simulink model "Aloe_E_Cell_Project_2016"  (R2016b)
settings: Solver=VariableStepAuto  StartTime=0.0  StopTime=0.14  RelTol=1e-3
undefined symbols (not defined in the file): D1, Delta
libraries: powerlib x218, powerlib_meascontrol x6, simulink x2
(part 2 of 2)

== system Aloe_E_Cell_Project_2016/Aloe E Battery Array/12 V Aloe E-Cell26 ==
  Constant : Constant  Value=4
  Constant1 : Constant  Value=24
  Controlled Current Source : powerlib/Electrical Sources/Controlled Current Source  Initialize=on  Source_Type=DC  Amplitude=1  Phase=0  Frequency=0  Measurements=None
  Controlled Voltage Source : powerlib/Electrical Sources/Controlled Voltage Source  Initialize=on  Source_Type=DC  Amplitude=1  Phase=0  Frequency=0  Measurements=Voltage
  Current Measurement : powerlib/Measurements/Current Measurement  PhasorSimulation=off  OutputType=Complex  PSBequivalent=0
  Display : Display
      settings: Decimation=3
  Display1 : Display
      settings: Decimation=3
  Series RLC Branch1 : powerlib/Elements/Series RLC Branch  LConnTagsString=__new0  RConnTagsString=__new0  BranchType=R  Resistance=6  Inductance=1e-3  SetiL0=off  InitialCurrent=0  Capacitance=1e-6  Setx0=off  InitialVoltage=0  Measurements=None
  Voltage Measurement : powerlib/Measurements/Voltage Measurement  PhasorSimulation=off  OutputType=Complex  PSBequivalent=0
  V+ : PMIOPort  Side=Right
  "V- " : PMIOPort  Port=2  Side=Right
  wires:
  Constant/1 -> Controlled Current Source/1
  Constant1/1 -> Controlled Voltage Source/1
  Current Measurement/1 -> Display1/1
  Voltage Measurement/1 -> Display/1
  connections:
  Series RLC Branch1/LConn1 -- Current Measurement/RConn1 -- Voltage Measurement/LConn1 -- V+/RConn1
  Controlled Voltage Source/RConn1 -- Controlled Current Source/LConn1
  Controlled Voltage Source/LConn1 -- Series RLC Branch1/RConn1 -- Voltage Measurement/LConn2 -- "V- "/RConn1
  Controlled Current Source/RConn1 -- Current Measurement/LConn1

== system Aloe_E_Cell_Project_2016/Aloe E Battery Array/12 V Aloe E-Cell27 ==
  Constant : Constant  Value=4
  Constant1 : Constant  Value=24
  Controlled Current Source : powerlib/Electrical Sources/Controlled Current Source  Initialize=on  Source_Type=DC  Amplitude=1  Phase=0  Frequency=0  Measurements=None
  Controlled Voltage Source : powerlib/Electrical Sources/Controlled Voltage Source  Initialize=on  Source_Type=DC  Amplitude=1  Phase=0  Frequency=0  Measurements=Voltage
  Current Measurement : powerlib/Measurements/Current Measurement  PhasorSimulation=off  OutputType=Complex  PSBequivalent=0
  Display : Display
      settings: Decimation=3
  Display1 : Display
      settings: Decimation=3
  Series RLC Branch1 : powerlib/Elements/Series RLC Branch  LConnTagsString=__new0  RConnTagsString=__new0  BranchType=R  Resistance=6  Inductance=1e-3  SetiL0=off  InitialCurrent=0  Capacitance=1e-6  Setx0=off  InitialVoltage=0  Measurements=None
  Voltage Measurement : powerlib/Measurements/Voltage Measurement  PhasorSimulation=off  OutputType=Complex  PSBequivalent=0
  V+ : PMIOPort  Side=Right
  "V- " : PMIOPort  Port=2  Side=Right
  wires:
  Voltage Measurement/1 -> Display/1
  Current Measurement/1 -> Display1/1
  Constant1/1 -> Controlled Voltage Source/1
  Constant/1 -> Controlled Current Source/1
  connections:
  Controlled Current Source/RConn1 -- Current Measurement/LConn1
  "V- "/RConn1 -- Voltage Measurement/LConn2 -- Series RLC Branch1/RConn1 -- Controlled Voltage Source/LConn1
  Controlled Voltage Source/RConn1 -- Controlled Current Source/LConn1
  V+/RConn1 -- Voltage Measurement/LConn1 -- Current Measurement/RConn1 -- Series RLC Branch1/LConn1

== system Aloe_E_Cell_Project_2016/Aloe E Battery Array/12 V Aloe E-Cell28 ==
  Constant : Constant  Value=4
  Constant1 : Constant  Value=24
  Controlled Current Source : powerlib/Electrical Sources/Controlled Current Source  Initialize=on  Source_Type=DC  Amplitude=1  Phase=0  Frequency=0  Measurements=None
  Controlled Voltage Source : powerlib/Electrical Sources/Controlled Voltage Source  Initialize=on  Source_Type=DC  Amplitude=1  Phase=0  Frequency=0  Measurements=Voltage
  Current Measurement : powerlib/Measurements/Current Measurement  PhasorSimulation=off  OutputType=Complex  PSBequivalent=0
  Display : Display
      settings: Decimation=3
  Display1 : Display
      settings: Decimation=3
  Series RLC Branch1 : powerlib/Elements/Series RLC Branch  LConnTagsString=__new0  RConnTagsString=__new0  BranchType=R  Resistance=6  Inductance=1e-3  SetiL0=off  InitialCurrent=0  Capacitance=1e-6  Setx0=off  InitialVoltage=0  Measurements=None
  Voltage Measurement : powerlib/Measurements/Voltage Measurement  PhasorSimulation=off  OutputType=Complex  PSBequivalent=0
  V+ : PMIOPort  Side=Right
  "V- " : PMIOPort  Port=2  Side=Right
  wires:
  Voltage Measurement/1 -> Display/1
  Current Measurement/1 -> Display1/1
  Constant1/1 -> Controlled Voltage Source/1
  Constant/1 -> Controlled Current Source/1
  connections:
  Controlled Current Source/RConn1 -- Current Measurement/LConn1
  "V- "/RConn1 -- Voltage Measurement/LConn2 -- Series RLC Branch1/RConn1 -- Controlled Voltage Source/LConn1
  Controlled Voltage Source/RConn1 -- Controlled Current Source/LConn1
  V+/RConn1 -- Voltage Measurement/LConn1 -- Current Measurement/RConn1 -- Series RLC Branch1/LConn1

== system Aloe_E_Cell_Project_2016/Aloe E Battery Array/12 V Aloe E-Cell29 ==
  Constant : Constant  Value=4
  Constant1 : Constant  Value=24
  Controlled Current Source : powerlib/Electrical Sources/Controlled Current Source  Initialize=on  Source_Type=DC  Amplitude=1  Phase=0  Frequency=0  Measurements=None
  Controlled Voltage Source : powerlib/Electrical Sources/Controlled Voltage Source  Initialize=on  Source_Type=DC  Amplitude=1  Phase=0  Frequency=0  Measurements=Voltage
  Current Measurement : powerlib/Measurements/Current Measurement  PhasorSimulation=off  OutputType=Complex  PSBequivalent=0
  Display : Display
      settings: Decimation=3
  Display1 : Display
      settings: Decimation=3
  Series RLC Branch1 : powerlib/Elements/Series RLC Branch  LConnTagsString=__new0  RConnTagsString=__new0  BranchType=R  Resistance=6  Inductance=1e-3  SetiL0=off  InitialCurrent=0  Capacitance=1e-6  Setx0=off  InitialVoltage=0  Measurements=None
  Voltage Measurement : powerlib/Measurements/Voltage Measurement  PhasorSimulation=off  OutputType=Complex  PSBequivalent=0
  V+ : PMIOPort  Side=Right
  "V- " : PMIOPort  Port=2  Side=Right
  wires:
  Constant/1 -> Controlled Current Source/1
  Constant1/1 -> Controlled Voltage Source/1
  Current Measurement/1 -> Display1/1
  Voltage Measurement/1 -> Display/1
  connections:
  Series RLC Branch1/LConn1 -- Current Measurement/RConn1 -- Voltage Measurement/LConn1 -- V+/RConn1
  Controlled Voltage Source/RConn1 -- Controlled Current Source/LConn1
  Controlled Voltage Source/LConn1 -- Series RLC Branch1/RConn1 -- Voltage Measurement/LConn2 -- "V- "/RConn1
  Controlled Current Source/RConn1 -- Current Measurement/LConn1

== system Aloe_E_Cell_Project_2016/Aloe E Battery Array/12 V Aloe E-Cell3 ==
  Constant : Constant  Value=4
  Constant1 : Constant  Value=24
  Controlled Current Source : powerlib/Electrical Sources/Controlled Current Source  Initialize=on  Source_Type=DC  Amplitude=1  Phase=0  Frequency=0  Measurements=None
  Controlled Voltage Source : powerlib/Electrical Sources/Controlled Voltage Source  Initialize=on  Source_Type=DC  Amplitude=1  Phase=0  Frequency=0  Measurements=Voltage
  Current Measurement : powerlib/Measurements/Current Measurement  PhasorSimulation=off  OutputType=Complex  PSBequivalent=0
  Display : Display
      settings: Decimation=3
  Display1 : Display
      settings: Decimation=3
  Series RLC Branch1 : powerlib/Elements/Series RLC Branch  LConnTagsString=__new0  RConnTagsString=__new0  BranchType=R  Resistance=6  Inductance=1e-3  SetiL0=off  InitialCurrent=0  Capacitance=1e-6  Setx0=off  InitialVoltage=0  Measurements=None
  Voltage Measurement : powerlib/Measurements/Voltage Measurement  PhasorSimulation=off  OutputType=Complex  PSBequivalent=0
  V+ : PMIOPort  Side=Right
  "V- " : PMIOPort  Port=2  Side=Right
  wires:
  Constant/1 -> Controlled Current Source/1
  Constant1/1 -> Controlled Voltage Source/1
  Current Measurement/1 -> Display1/1
  Voltage Measurement/1 -> Display/1
  connections:
  Series RLC Branch1/LConn1 -- Current Measurement/RConn1 -- Voltage Measurement/LConn1 -- V+/RConn1
  Controlled Voltage Source/RConn1 -- Controlled Current Source/LConn1
  Controlled Voltage Source/LConn1 -- Series RLC Branch1/RConn1 -- Voltage Measurement/LConn2 -- "V- "/RConn1
  Controlled Current Source/RConn1 -- Current Measurement/LConn1

== system Aloe_E_Cell_Project_2016/Aloe E Battery Array/12 V Aloe E-Cell30 ==
  Constant : Constant  Value=4
  Constant1 : Constant  Value=24
  Controlled Current Source : powerlib/Electrical Sources/Controlled Current Source  Initialize=on  Source_Type=DC  Amplitude=1  Phase=0  Frequency=0  Measurements=None
  Controlled Voltage Source : powerlib/Electrical Sources/Controlled Voltage Source  Initialize=on  Source_Type=DC  Amplitude=1  Phase=0  Frequency=0  Measurements=Voltage
  Current Measurement : powerlib/Measurements/Current Measurement  PhasorSimulation=off  OutputType=Complex  PSBequivalent=0
  Display : Display
      settings: Decimation=3
  Display1 : Display
      settings: Decimation=3
  Series RLC Branch1 : powerlib/Elements/Series RLC Branch  LConnTagsString=__new0  RConnTagsString=__new0  BranchType=R  Resistance=6  Inductance=1e-3  SetiL0=off  InitialCurrent=0  Capacitance=1e-6  Setx0=off  InitialVoltage=0  Measurements=None
  Voltage Measurement : powerlib/Measurements/Voltage Measurement  PhasorSimulation=off  OutputType=Complex  PSBequivalent=0
  V+ : PMIOPort  Side=Right
  "V- " : PMIOPort  Port=2  Side=Right
  wires:
  Constant/1 -> Controlled Current Source/1
  Constant1/1 -> Controlled Voltage Source/1
  Current Measurement/1 -> Display1/1
  Voltage Measurement/1 -> Display/1
  connections:
  Series RLC Branch1/LConn1 -- Current Measurement/RConn1 -- Voltage Measurement/LConn1 -- V+/RConn1
  Controlled Voltage Source/RConn1 -- Controlled Current Source/LConn1
  Controlled Voltage Source/LConn1 -- Series RLC Branch1/RConn1 -- Voltage Measurement/LConn2 -- "V- "/RConn1
  Controlled Current Source/RConn1 -- Current Measurement/LConn1

== system Aloe_E_Cell_Project_2016/Aloe E Battery Array/12 V Aloe E-Cell31 ==
  Constant : Constant  Value=4
  Constant1 : Constant  Value=24
  Controlled Current Source : powerlib/Electrical Sources/Controlled Current Source  Initialize=on  Source_Type=DC  Amplitude=1  Phase=0  Frequency=0  Measurements=None
  Controlled Voltage Source : powerlib/Electrical Sources/Controlled Voltage Source  Initialize=on  Source_Type=DC  Amplitude=1  Phase=0  Frequency=0  Measurements=Voltage
  Current Measurement : powerlib/Measurements/Current Measurement  PhasorSimulation=off  OutputType=Complex  PSBequivalent=0
  Display : Display
      settings: Decimation=3
  Display1 : Display
      settings: Decimation=3
  Series RLC Branch1 : powerlib/Elements/Series RLC Branch  LConnTagsString=__new0  RConnTagsString=__new0  BranchType=R  Resistance=6  Inductance=1e-3  SetiL0=off  InitialCurrent=0  Capacitance=1e-6  Setx0=off  InitialVoltage=0  Measurements=None
  Voltage Measurement : powerlib/Measurements/Voltage Measurement  PhasorSimulation=off  OutputType=Complex  PSBequivalent=0
  V+ : PMIOPort  Side=Right
  "V- " : PMIOPort  Port=2  Side=Right
  wires:
  Voltage Measurement/1 -> Display/1
  Current Measurement/1 -> Display1/1
  Constant1/1 -> Controlled Voltage Source/1
  Constant/1 -> Controlled Current Source/1
  connections:
  Controlled Current Source/RConn1 -- Current Measurement/LConn1
  "V- "/RConn1 -- Voltage Measurement/LConn2 -- Series RLC Branch1/RConn1 -- Controlled Voltage Source/LConn1
  Controlled Voltage Source/RConn1 -- Controlled Current Source/LConn1
  V+/RConn1 -- Voltage Measurement/LConn1 -- Current Measurement/RConn1 -- Series RLC Branch1/LConn1

== system Aloe_E_Cell_Project_2016/Aloe E Battery Array/12 V Aloe E-Cell32 ==
  Constant : Constant  Value=4
  Constant1 : Constant  Value=24
  Controlled Current Source : powerlib/Electrical Sources/Controlled Current Source  Initialize=on  Source_Type=DC  Amplitude=1  Phase=0  Frequency=0  Measurements=None
  Controlled Voltage Source : powerlib/Electrical Sources/Controlled Voltage Source  Initialize=on  Source_Type=DC  Amplitude=1  Phase=0  Frequency=0  Measurements=Voltage
  Current Measurement : powerlib/Measurements/Current Measurement  PhasorSimulation=off  OutputType=Complex  PSBequivalent=0
  Display : Display
      settings: Decimation=3
  Display1 : Display
      settings: Decimation=3
  Series RLC Branch1 : powerlib/Elements/Series RLC Branch  LConnTagsString=__new0  RConnTagsString=__new0  BranchType=R  Resistance=6  Inductance=1e-3  SetiL0=off  InitialCurrent=0  Capacitance=1e-6  Setx0=off  InitialVoltage=0  Measurements=None
  Voltage Measurement : powerlib/Measurements/Voltage Measurement  PhasorSimulation=off  OutputType=Complex  PSBequivalent=0
  V+ : PMIOPort  Side=Right
  "V- " : PMIOPort  Port=2  Side=Right
  wires:
  Constant/1 -> Controlled Current Source/1
  Constant1/1 -> Controlled Voltage Source/1
  Current Measurement/1 -> Display1/1
  Voltage Measurement/1 -> Display/1
  connections:
  Series RLC Branch1/LConn1 -- Current Measurement/RConn1 -- Voltage Measurement/LConn1 -- V+/RConn1
  Controlled Voltage Source/RConn1 -- Controlled Current Source/LConn1
  Controlled Voltage Source/LConn1 -- Series RLC Branch1/RConn1 -- Voltage Measurement/LConn2 -- "V- "/RConn1
  Controlled Current Source/RConn1 -- Current Measurement/LConn1

== system Aloe_E_Cell_Project_2016/Aloe E Battery Array/12 V Aloe E-Cell33 ==
  Constant : Constant  Value=4
  Constant1 : Constant  Value=24
  Controlled Current Source : powerlib/Electrical Sources/Controlled Current Source  Initialize=on  Source_Type=DC  Amplitude=1  Phase=0  Frequency=0  Measurements=None
  Controlled Voltage Source : powerlib/Electrical Sources/Controlled Voltage Source  Initialize=on  Source_Type=DC  Amplitude=1  Phase=0  Frequency=0  Measurements=Voltage
  Current Measurement : powerlib/Measurements/Current Measurement  PhasorSimulation=off  OutputType=Complex  PSBequivalent=0
  Display : Display
      settings: Decimation=3
  Display1 : Display
      settings: Decimation=3
  Series RLC Branch1 : powerlib/Elements/Series RLC Branch  LConnTagsString=__new0  RConnTagsString=__new0  BranchType=R  Resistance=6  Inductance=1e-3  SetiL0=off  InitialCurrent=0  Capacitance=1e-6  Setx0=off  InitialVoltage=0  Measurements=None
  Voltage Measurement : powerlib/Measurements/Voltage Measurement  PhasorSimulation=off  OutputType=Complex  PSBequivalent=0
  V+ : PMIOPort  Side=Right
  "V- " : PMIOPort  Port=2  Side=Right
  wires:
  Constant/1 -> Controlled Current Source/1
  Constant1/1 -> Controlled Voltage Source/1
  Current Measurement/1 -> Display1/1
  Voltage Measurement/1 -> Display/1
  connections:
  Series RLC Branch1/LConn1 -- Current Measurement/RConn1 -- Voltage Measurement/LConn1 -- V+/RConn1
  Controlled Voltage Source/RConn1 -- Controlled Current Source/LConn1
  Controlled Voltage Source/LConn1 -- Series RLC Branch1/RConn1 -- Voltage Measurement/LConn2 -- "V- "/RConn1
  Controlled Current Source/RConn1 -- Current Measurement/LConn1

== system Aloe_E_Cell_Project_2016/Aloe E Battery Array/12 V Aloe E-Cell34 ==
  Constant : Constant  Value=4
  Constant1 : Constant  Value=24
  Controlled Current Source : powerlib/Electrical Sources/Controlled Current Source  Initialize=on  Source_Type=DC  Amplitude=1  Phase=0  Frequency=0  Measurements=None
  Controlled Voltage Source : powerlib/Electrical Sources/Controlled Voltage Source  Initialize=on  Source_Type=DC  Amplitude=1  Phase=0  Frequency=0  Measurements=Voltage
  Current Measurement : powerlib/Measurements/Current Measurement  PhasorSimulation=off  OutputType=Complex  PSBequivalent=0
  Display : Display
      settings: Decimation=3
  Display1 : Display
      settings: Decimation=3
  Series RLC Branch1 : powerlib/Elements/Series RLC Branch  LConnTagsString=__new0  RConnTagsString=__new0  BranchType=R  Resistance=6  Inductance=1e-3  SetiL0=off  InitialCurrent=0  Capacitance=1e-6  Setx0=off  InitialVoltage=0  Measurements=None
  Voltage Measurement : powerlib/Measurements/Voltage Measurement  PhasorSimulation=off  OutputType=Complex  PSBequivalent=0
  V+ : PMIOPort  Side=Right
  "V- " : PMIOPort  Port=2  Side=Right
  wires:
  Voltage Measurement/1 -> Display/1
  Current Measurement/1 -> Display1/1
  Constant1/1 -> Controlled Voltage Source/1
  Constant/1 -> Controlled Current Source/1
  connections:
  Controlled Current Source/RConn1 -- Current Measurement/LConn1
  "V- "/RConn1 -- Voltage Measurement/LConn2 -- Series RLC Branch1/RConn1 -- Controlled Voltage Source/LConn1
  Controlled Voltage Source/RConn1 -- Controlled Current Source/LConn1
  V+/RConn1 -- Voltage Measurement/LConn1 -- Current Measurement/RConn1 -- Series RLC Branch1/LConn1

== system Aloe_E_Cell_Project_2016/Aloe E Battery Array/12 V Aloe E-Cell35 ==
  Constant : Constant  Value=4
  Constant1 : Constant  Value=24
  Controlled Current Source : powerlib/Electrical Sources/Controlled Current Source  Initialize=on  Source_Type=DC  Amplitude=1  Phase=0  Frequency=0  Measurements=None
  Controlled Voltage Source : powerlib/Electrical Sources/Controlled Voltage Source  Initialize=on  Source_Type=DC  Amplitude=1  Phase=0  Frequency=0  Measurements=Voltage
  Current Measurement : powerlib/Measurements/Current Measurement  PhasorSimulation=off  OutputType=Complex  PSBequivalent=0
  Display : Display
      settings: Decimation=3
  Display1 : Display
      settings: Decimation=3
  Series RLC Branch1 : powerlib/Elements/Series RLC Branch  LConnTagsString=__new0  RConnTagsString=__new0  BranchType=R  Resistance=6  Inductance=1e-3  SetiL0=off  InitialCurrent=0  Capacitance=1e-6  Setx0=off  InitialVoltage=0  Measurements=None
  Voltage Measurement : powerlib/Measurements/Voltage Measurement  PhasorSimulation=off  OutputType=Complex  PSBequivalent=0
  V+ : PMIOPort  Side=Right
  "V- " : PMIOPort  Port=2  Side=Right
  wires:
  Constant/1 -> Controlled Current Source/1
  Constant1/1 -> Controlled Voltage Source/1
  Current Measurement/1 -> Display1/1
  Voltage Measurement/1 -> Display/1
  connections:
  Series RLC Branch1/LConn1 -- Current Measurement/RConn1 -- Voltage Measurement/LConn1 -- V+/RConn1
  Controlled Voltage Source/RConn1 -- Controlled Current Source/LConn1
  Controlled Voltage Source/LConn1 -- Series RLC Branch1/RConn1 -- Voltage Measurement/LConn2 -- "V- "/RConn1
  Controlled Current Source/RConn1 -- Current Measurement/LConn1

== system Aloe_E_Cell_Project_2016/Aloe E Battery Array/12 V Aloe E-Cell36 ==
  Constant : Constant  Value=4
  Constant1 : Constant  Value=24
  Controlled Current Source : powerlib/Electrical Sources/Controlled Current Source  Initialize=on  Source_Type=DC  Amplitude=1  Phase=0  Frequency=0  Measurements=None
  Controlled Voltage Source : powerlib/Electrical Sources/Controlled Voltage Source  Initialize=on  Source_Type=DC  Amplitude=1  Phase=0  Frequency=0  Measurements=Voltage
  Current Measurement : powerlib/Measurements/Current Measurement  PhasorSimulation=off  OutputType=Complex  PSBequivalent=0
  Display : Display
      settings: Decimation=3
  Display1 : Display
      settings: Decimation=3
  Series RLC Branch1 : powerlib/Elements/Series RLC Branch  LConnTagsString=__new0  RConnTagsString=__new0  BranchType=R  Resistance=6  Inductance=1e-3  SetiL0=off  InitialCurrent=0  Capacitance=1e-6  Setx0=off  InitialVoltage=0  Measurements=None
  Voltage Measurement : powerlib/Measurements/Voltage Measurement  PhasorSimulation=off  OutputType=Complex  PSBequivalent=0
  V+ : PMIOPort  Side=Right
  "V- " : PMIOPort  Port=2  Side=Right
  wires:
  Constant/1 -> Controlled Current Source/1
  Constant1/1 -> Controlled Voltage Source/1
  Current Measurement/1 -> Display1/1
  Voltage Measurement/1 -> Display/1
  connections:
  Series RLC Branch1/LConn1 -- Current Measurement/RConn1 -- Voltage Measurement/LConn1 -- V+/RConn1
  Controlled Voltage Source/RConn1 -- Controlled Current Source/LConn1
  Controlled Voltage Source/LConn1 -- Series RLC Branch1/RConn1 -- Voltage Measurement/LConn2 -- "V- "/RConn1
  Controlled Current Source/RConn1 -- Current Measurement/LConn1

== system Aloe_E_Cell_Project_2016/Aloe E Battery Array/12 V Aloe E-Cell37 ==
  Constant : Constant  Value=4
  Constant1 : Constant  Value=24
  Controlled Current Source : powerlib/Electrical Sources/Controlled Current Source  Initialize=on  Source_Type=DC  Amplitude=1  Phase=0  Frequency=0  Measurements=None
  Controlled Voltage Source : powerlib/Electrical Sources/Controlled Voltage Source  Initialize=on  Source_Type=DC  Amplitude=1  Phase=0  Frequency=0  Measurements=Voltage
  Current Measurement : powerlib/Measurements/Current Measurement  PhasorSimulation=off  OutputType=Complex  PSBequivalent=0
  Display : Display
      settings: Decimation=3
  Display1 : Display
      settings: Decimation=3
  Series RLC Branch1 : powerlib/Elements/Series RLC Branch  LConnTagsString=__new0  RConnTagsString=__new0  BranchType=R  Resistance=6  Inductance=1e-3  SetiL0=off  InitialCurrent=0  Capacitance=1e-6  Setx0=off  InitialVoltage=0  Measurements=None
  Voltage Measurement : powerlib/Measurements/Voltage Measurement  PhasorSimulation=off  OutputType=Complex  PSBequivalent=0
  V+ : PMIOPort  Side=Right
  "V- " : PMIOPort  Port=2  Side=Right
  wires:
  Voltage Measurement/1 -> Display/1
  Current Measurement/1 -> Display1/1
  Constant1/1 -> Controlled Voltage Source/1
  Constant/1 -> Controlled Current Source/1
  connections:
  Controlled Current Source/RConn1 -- Current Measurement/LConn1
  "V- "/RConn1 -- Voltage Measurement/LConn2 -- Series RLC Branch1/RConn1 -- Controlled Voltage Source/LConn1
  Controlled Voltage Source/RConn1 -- Controlled Current Source/LConn1
  V+/RConn1 -- Voltage Measurement/LConn1 -- Current Measurement/RConn1 -- Series RLC Branch1/LConn1

== system Aloe_E_Cell_Project_2016/Aloe E Battery Array/12 V Aloe E-Cell38 ==
  Constant : Constant  Value=4
  Constant1 : Constant  Value=24
  Controlled Current Source : powerlib/Electrical Sources/Controlled Current Source  Initialize=on  Source_Type=DC  Amplitude=1  Phase=0  Frequency=0  Measurements=None
  Controlled Voltage Source : powerlib/Electrical Sources/Controlled Voltage Source  Initialize=on  Source_Type=DC  Amplitude=1  Phase=0  Frequency=0  Measurements=Voltage
  Current Measurement : powerlib/Measurements/Current Measurement  PhasorSimulation=off  OutputType=Complex  PSBequivalent=0
  Display : Display
      settings: Decimation=3
  Display1 : Display
      settings: Decimation=3
  Series RLC Branch1 : powerlib/Elements/Series RLC Branch  LConnTagsString=__new0  RConnTagsString=__new0  BranchType=R  Resistance=6  Inductance=1e-3  SetiL0=off  InitialCurrent=0  Capacitance=1e-6  Setx0=off  InitialVoltage=0  Measurements=None
  Voltage Measurement : powerlib/Measurements/Voltage Measurement  PhasorSimulation=off  OutputType=Complex  PSBequivalent=0
  V+ : PMIOPort  Side=Right
  "V- " : PMIOPort  Port=2  Side=Right
  wires:
  Voltage Measurement/1 -> Display/1
  Current Measurement/1 -> Display1/1
  Constant1/1 -> Controlled Voltage Source/1
  Constant/1 -> Controlled Current Source/1
  connections:
  Controlled Current Source/RConn1 -- Current Measurement/LConn1
  "V- "/RConn1 -- Voltage Measurement/LConn2 -- Series RLC Branch1/RConn1 -- Controlled Voltage Source/LConn1
  Controlled Voltage Source/RConn1 -- Controlled Current Source/LConn1
  V+/RConn1 -- Voltage Measurement/LConn1 -- Current Measurement/RConn1 -- Series RLC Branch1/LConn1

== system Aloe_E_Cell_Project_2016/Aloe E Battery Array/12 V Aloe E-Cell39 ==
  Constant : Constant  Value=4
  Constant1 : Constant  Value=24
  Controlled Current Source : powerlib/Electrical Sources/Controlled Current Source  Initialize=on  Source_Type=DC  Amplitude=1  Phase=0  Frequency=0  Measurements=None
  Controlled Voltage Source : powerlib/Electrical Sources/Controlled Voltage Source  Initialize=on  Source_Type=DC  Amplitude=1  Phase=0  Frequency=0  Measurements=Voltage
  Current Measurement : powerlib/Measurements/Current Measurement  PhasorSimulation=off  OutputType=Complex  PSBequivalent=0
  Display : Display
      settings: Decimation=3
  Display1 : Display
      settings: Decimation=3
  Series RLC Branch1 : powerlib/Elements/Series RLC Branch  LConnTagsString=__new0  RConnTagsString=__new0  BranchType=R  Resistance=6  Inductance=1e-3  SetiL0=off  InitialCurrent=0  Capacitance=1e-6  Setx0=off  InitialVoltage=0  Measurements=None
  Voltage Measurement : powerlib/Measurements/Voltage Measurement  PhasorSimulation=off  OutputType=Complex  PSBequivalent=0
  V+ : PMIOPort  Side=Right
  "V- " : PMIOPort  Port=2  Side=Right
  wires:
  Constant/1 -> Controlled Current Source/1
  Constant1/1 -> Controlled Voltage Source/1
  Current Measurement/1 -> Display1/1
  Voltage Measurement/1 -> Display/1
  connections:
  Series RLC Branch1/LConn1 -- Current Measurement/RConn1 -- Voltage Measurement/LConn1 -- V+/RConn1
  Controlled Voltage Source/RConn1 -- Controlled Current Source/LConn1
  Controlled Voltage Source/LConn1 -- Series RLC Branch1/RConn1 -- Voltage Measurement/LConn2 -- "V- "/RConn1
  Controlled Current Source/RConn1 -- Current Measurement/LConn1

== system Aloe_E_Cell_Project_2016/Aloe E Battery Array/12 V Aloe E-Cell4 ==
  Constant : Constant  Value=4
  Constant1 : Constant  Value=24
  Controlled Current Source : powerlib/Electrical Sources/Controlled Current Source  Initialize=on  Source_Type=DC  Amplitude=1  Phase=0  Frequency=0  Measurements=None
  Controlled Voltage Source : powerlib/Electrical Sources/Controlled Voltage Source  Initialize=on  Source_Type=DC  Amplitude=1  Phase=0  Frequency=0  Measurements=Voltage
  Current Measurement : powerlib/Measurements/Current Measurement  PhasorSimulation=off  OutputType=Complex  PSBequivalent=0
  Display : Display
      settings: Decimation=3
  Display1 : Display
      settings: Decimation=3
  Series RLC Branch1 : powerlib/Elements/Series RLC Branch  LConnTagsString=__new0  RConnTagsString=__new0  BranchType=R  Resistance=6  Inductance=1e-3  SetiL0=off  InitialCurrent=0  Capacitance=1e-6  Setx0=off  InitialVoltage=0  Measurements=None
  Voltage Measurement : powerlib/Measurements/Voltage Measurement  PhasorSimulation=off  OutputType=Complex  PSBequivalent=0
  V+ : PMIOPort  Side=Right
  "V- " : PMIOPort  Port=2  Side=Right
  wires:
  Voltage Measurement/1 -> Display/1
  Current Measurement/1 -> Display1/1
  Constant1/1 -> Controlled Voltage Source/1
  Constant/1 -> Controlled Current Source/1
  connections:
  Controlled Current Source/RConn1 -- Current Measurement/LConn1
  "V- "/RConn1 -- Voltage Measurement/LConn2 -- Series RLC Branch1/RConn1 -- Controlled Voltage Source/LConn1
  Controlled Voltage Source/RConn1 -- Controlled Current Source/LConn1
  V+/RConn1 -- Voltage Measurement/LConn1 -- Current Measurement/RConn1 -- Series RLC Branch1/LConn1

== system Aloe_E_Cell_Project_2016/Aloe E Battery Array/12 V Aloe E-Cell40 ==
  Constant : Constant  Value=4
  Constant1 : Constant  Value=24
  Controlled Current Source : powerlib/Electrical Sources/Controlled Current Source  Initialize=on  Source_Type=DC  Amplitude=1  Phase=0  Frequency=0  Measurements=None
  Controlled Voltage Source : powerlib/Electrical Sources/Controlled Voltage Source  Initialize=on  Source_Type=DC  Amplitude=1  Phase=0  Frequency=0  Measurements=Voltage
  Current Measurement : powerlib/Measurements/Current Measurement  PhasorSimulation=off  OutputType=Complex  PSBequivalent=0
  Display : Display
      settings: Decimation=3
  Display1 : Display
      settings: Decimation=3
  Series RLC Branch1 : powerlib/Elements/Series RLC Branch  LConnTagsString=__new0  RConnTagsString=__new0  BranchType=R  Resistance=6  Inductance=1e-3  SetiL0=off  InitialCurrent=0  Capacitance=1e-6  Setx0=off  InitialVoltage=0  Measurements=None
  Voltage Measurement : powerlib/Measurements/Voltage Measurement  PhasorSimulation=off  OutputType=Complex  PSBequivalent=0
  V+ : PMIOPort  Side=Right
  "V- " : PMIOPort  Port=2  Side=Right
  wires:
  Voltage Measurement/1 -> Display/1
  Current Measurement/1 -> Display1/1
  Constant1/1 -> Controlled Voltage Source/1
  Constant/1 -> Controlled Current Source/1
  connections:
  Controlled Current Source/RConn1 -- Current Measurement/LConn1
  "V- "/RConn1 -- Voltage Measurement/LConn2 -- Series RLC Branch1/RConn1 -- Controlled Voltage Source/LConn1
  Controlled Voltage Source/RConn1 -- Controlled Current Source/LConn1
  V+/RConn1 -- Voltage Measurement/LConn1 -- Current Measurement/RConn1 -- Series RLC Branch1/LConn1

== system Aloe_E_Cell_Project_2016/Aloe E Battery Array/12 V Aloe E-Cell5 ==
  Constant : Constant  Value=4
  Constant1 : Constant  Value=24
  Controlled Current Source : powerlib/Electrical Sources/Controlled Current Source  Initialize=on  Source_Type=DC  Amplitude=1  Phase=0  Frequency=0  Measurements=None
  Controlled Voltage Source : powerlib/Electrical Sources/Controlled Voltage Source  Initialize=on  Source_Type=DC  Amplitude=1  Phase=0  Frequency=0  Measurements=Voltage
  Current Measurement : powerlib/Measurements/Current Measurement  PhasorSimulation=off  OutputType=Complex  PSBequivalent=0
  Display : Display
      settings: Decimation=3
  Display1 : Display
      settings: Decimation=3
  Series RLC Branch1 : powerlib/Elements/Series RLC Branch  LConnTagsString=__new0  RConnTagsString=__new0  BranchType=R  Resistance=6  Inductance=1e-3  SetiL0=off  InitialCurrent=0  Capacitance=1e-6  Setx0=off  InitialVoltage=0  Measurements=None
  Voltage Measurement : powerlib/Measurements/Voltage Measurement  PhasorSimulation=off  OutputType=Complex  PSBequivalent=0
  V+ : PMIOPort  Side=Right
  "V- " : PMIOPort  Port=2  Side=Right
  wires:
  Voltage Measurement/1 -> Display/1
  Current Measurement/1 -> Display1/1
  Constant1/1 -> Controlled Voltage Source/1
  Constant/1 -> Controlled Current Source/1
  connections:
  Controlled Current Source/RConn1 -- Current Measurement/LConn1
  "V- "/RConn1 -- Voltage Measurement/LConn2 -- Series RLC Branch1/RConn1 -- Controlled Voltage Source/LConn1
  Controlled Voltage Source/RConn1 -- Controlled Current Source/LConn1
  V+/RConn1 -- Voltage Measurement/LConn1 -- Current Measurement/RConn1 -- Series RLC Branch1/LConn1

== system Aloe_E_Cell_Project_2016/Aloe E Battery Array/12 V Aloe E-Cell6 ==
  Constant : Constant  Value=4
  Constant1 : Constant  Value=24
  Controlled Current Source : powerlib/Electrical Sources/Controlled Current Source  Initialize=on  Source_Type=DC  Amplitude=1  Phase=0  Frequency=0  Measurements=None
  Controlled Voltage Source : powerlib/Electrical Sources/Controlled Voltage Source  Initialize=on  Source_Type=DC  Amplitude=1  Phase=0  Frequency=0  Measurements=Voltage
  Current Measurement : powerlib/Measurements/Current Measurement  PhasorSimulation=off  OutputType=Complex  PSBequivalent=0
  Display : Display
      settings: Decimation=3
  Display1 : Display
      settings: Decimation=3
  Series RLC Branch1 : powerlib/Elements/Series RLC Branch  LConnTagsString=__new0  RConnTagsString=__new0  BranchType=R  Resistance=6  Inductance=1e-3  SetiL0=off  InitialCurrent=0  Capacitance=1e-6  Setx0=off  InitialVoltage=0  Measurements=None
  Voltage Measurement : powerlib/Measurements/Voltage Measurement  PhasorSimulation=off  OutputType=Complex  PSBequivalent=0
  V+ : PMIOPort  Side=Right
  "V- " : PMIOPort  Port=2  Side=Right
  wires:
  Constant/1 -> Controlled Current Source/1
  Constant1/1 -> Controlled Voltage Source/1
  Current Measurement/1 -> Display1/1
  Voltage Measurement/1 -> Display/1
  connections:
  Series RLC Branch1/LConn1 -- Current Measurement/RConn1 -- Voltage Measurement/LConn1 -- V+/RConn1
  Controlled Voltage Source/RConn1 -- Controlled Current Source/LConn1
  Controlled Voltage Source/LConn1 -- Series RLC Branch1/RConn1 -- Voltage Measurement/LConn2 -- "V- "/RConn1
  Controlled Current Source/RConn1 -- Current Measurement/LConn1

== system Aloe_E_Cell_Project_2016/Aloe E Battery Array/12 V Aloe E-Cell7 ==
  Constant : Constant  Value=4
  Constant1 : Constant  Value=24
  Controlled Current Source : powerlib/Electrical Sources/Controlled Current Source  Initialize=on  Source_Type=DC  Amplitude=1  Phase=0  Frequency=0  Measurements=None
  Controlled Voltage Source : powerlib/Electrical Sources/Controlled Voltage Source  Initialize=on  Source_Type=DC  Amplitude=1  Phase=0  Frequency=0  Measurements=Voltage
  Current Measurement : powerlib/Measurements/Current Measurement  PhasorSimulation=off  OutputType=Complex  PSBequivalent=0
  Display : Display
      settings: Decimation=3
  Display1 : Display
      settings: Decimation=3
  Series RLC Branch1 : powerlib/Elements/Series RLC Branch  LConnTagsString=__new0  RConnTagsString=__new0  BranchType=R  Resistance=6  Inductance=1e-3  SetiL0=off  InitialCurrent=0  Capacitance=1e-6  Setx0=off  InitialVoltage=0  Measurements=None
  Voltage Measurement : powerlib/Measurements/Voltage Measurement  PhasorSimulation=off  OutputType=Complex  PSBequivalent=0
  V+ : PMIOPort  Side=Right
  "V- " : PMIOPort  Port=2  Side=Right
  wires:
  Constant/1 -> Controlled Current Source/1
  Constant1/1 -> Controlled Voltage Source/1
  Current Measurement/1 -> Display1/1
  Voltage Measurement/1 -> Display/1
  connections:
  Series RLC Branch1/LConn1 -- Current Measurement/RConn1 -- Voltage Measurement/LConn1 -- V+/RConn1
  Controlled Voltage Source/RConn1 -- Controlled Current Source/LConn1
  Controlled Voltage Source/LConn1 -- Series RLC Branch1/RConn1 -- Voltage Measurement/LConn2 -- "V- "/RConn1
  Controlled Current Source/RConn1 -- Current Measurement/LConn1

== system Aloe_E_Cell_Project_2016/Aloe E Battery Array/12 V Aloe E-Cell8 ==
  Constant : Constant  Value=4
  Constant1 : Constant  Value=24
  Controlled Current Source : powerlib/Electrical Sources/Controlled Current Source  Initialize=on  Source_Type=DC  Amplitude=1  Phase=0  Frequency=0  Measurements=None
  Controlled Voltage Source : powerlib/Electrical Sources/Controlled Voltage Source  Initialize=on  Source_Type=DC  Amplitude=1  Phase=0  Frequency=0  Measurements=Voltage
  Current Measurement : powerlib/Measurements/Current Measurement  PhasorSimulation=off  OutputType=Complex  PSBequivalent=0
  Display : Display
      settings: Decimation=3
  Display1 : Display
      settings: Decimation=3
  Series RLC Branch1 : powerlib/Elements/Series RLC Branch  LConnTagsString=__new0  RConnTagsString=__new0  BranchType=R  Resistance=6  Inductance=1e-3  SetiL0=off  InitialCurrent=0  Capacitance=1e-6  Setx0=off  InitialVoltage=0  Measurements=None
  Voltage Measurement : powerlib/Measurements/Voltage Measurement  PhasorSimulation=off  OutputType=Complex  PSBequivalent=0
  V+ : PMIOPort  Side=Right
  "V- " : PMIOPort  Port=2  Side=Right
  wires:
  Voltage Measurement/1 -> Display/1
  Current Measurement/1 -> Display1/1
  Constant1/1 -> Controlled Voltage Source/1
  Constant/1 -> Controlled Current Source/1
  connections:
  Controlled Current Source/RConn1 -- Current Measurement/LConn1
  "V- "/RConn1 -- Voltage Measurement/LConn2 -- Series RLC Branch1/RConn1 -- Controlled Voltage Source/LConn1
  Controlled Voltage Source/RConn1 -- Controlled Current Source/LConn1
  V+/RConn1 -- Voltage Measurement/LConn1 -- Current Measurement/RConn1 -- Series RLC Branch1/LConn1

== system Aloe_E_Cell_Project_2016/Aloe E Battery Array/12 V Aloe E-Cell9 ==
  Constant : Constant  Value=4
  Constant1 : Constant  Value=24
  Controlled Current Source : powerlib/Electrical Sources/Controlled Current Source  Initialize=on  Source_Type=DC  Amplitude=1  Phase=0  Frequency=0  Measurements=None
  Controlled Voltage Source : powerlib/Electrical Sources/Controlled Voltage Source  Initialize=on  Source_Type=DC  Amplitude=1  Phase=0  Frequency=0  Measurements=Voltage
  Current Measurement : powerlib/Measurements/Current Measurement  PhasorSimulation=off  OutputType=Complex  PSBequivalent=0
  Display : Display
      settings: Decimation=3
  Display1 : Display
      settings: Decimation=3
  Series RLC Branch1 : powerlib/Elements/Series RLC Branch  LConnTagsString=__new0  RConnTagsString=__new0  BranchType=R  Resistance=6  Inductance=1e-3  SetiL0=off  InitialCurrent=0  Capacitance=1e-6  Setx0=off  InitialVoltage=0  Measurements=None
  Voltage Measurement : powerlib/Measurements/Voltage Measurement  PhasorSimulation=off  OutputType=Complex  PSBequivalent=0
  V+ : PMIOPort  Side=Right
  "V- " : PMIOPort  Port=2  Side=Right
  wires:
  Constant/1 -> Controlled Current Source/1
  Constant1/1 -> Controlled Voltage Source/1
  Current Measurement/1 -> Display1/1
  Voltage Measurement/1 -> Display/1
  connections:
  Series RLC Branch1/LConn1 -- Current Measurement/RConn1 -- Voltage Measurement/LConn1 -- V+/RConn1
  Controlled Voltage Source/RConn1 -- Controlled Current Source/LConn1
  Controlled Voltage Source/LConn1 -- Series RLC Branch1/RConn1 -- Voltage Measurement/LConn2 -- "V- "/RConn1
  Controlled Current Source/RConn1 -- Current Measurement/LConn1

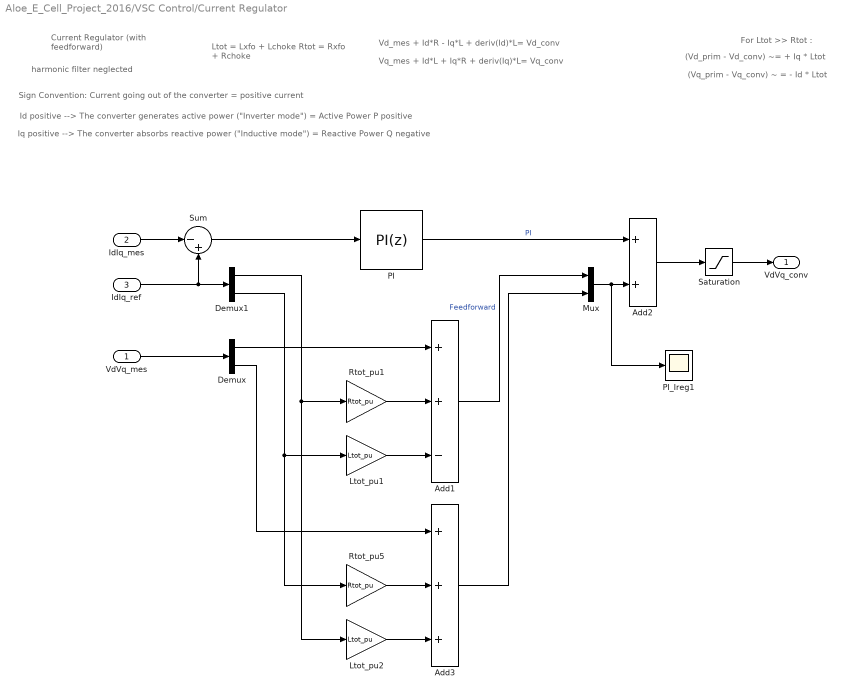
== system Aloe_E_Cell_Project_2016/VSC Control/Current Regulator ==
  note: harmonic filter neglected
  note: Vd_mes + Id*R - Iq*L + deriv(Id)*L= Vd_conv
  note: Vq_mes + Id*L + Iq*R + deriv(Iq)*L= Vq_conv
  note: Current Regulator
      | (with feedforward)
  note: Sign Convention: Current going out of the converter = positive current
  note: Iq positive --> The converter absorbs reactive power ("Inductive mode") = Reactive Power Q negative
  note: Id positive --> The converter generates active power ("Inverter mode") = Active Power P positive
  note: Ltot = Lxfo + Lchoke
      | Rtot = Rxfo + Rchoke
  note: (Vd_prim - Vd_conv) ~= + Iq * Ltot
  note: (Vq_prim - Vq_conv) ~ = - Id * Ltot
  note: For Ltot >> Rtot :
  VdVq_mes : Inport  PortDimensions=2
  IdIq_mes : Inport  Port=2  PortDimensions=2
  IdIq_ref : Inport  Port=3  PortDimensions=2
  Add1 : Sum  Inputs=++-
  Add2 : Sum
  Add3 : Sum  Inputs=+++
  Demux : Demux  Outputs=2
  Demux1 : Demux  Outputs=2
  Ltot_pu1 : Gain  Gain=Ltot_pu  SaturateOnIntegerOverflow=on  OutDataTypeStr=Inherit: Same as input  ParamDataTypeStr=Inherit: Same as input
  Ltot_pu2 : Gain  Gain=Ltot_pu  SaturateOnIntegerOverflow=on  OutDataTypeStr=Inherit: Same as input  ParamDataTypeStr=Inherit: Same as input
  Mux : Mux  Inputs=2
  PI : simulink/Continuous/PID Controller  Controller=PI  Form=Parallel  TimeDomain=Discrete-time  SampleTime=Ts  IntegratorMethod=Forward Euler  FilterMethod=Forward Euler  ControllerParametersSource=internal  P=Kp_Ireg  I=Ki_Ireg  D=0  UseFilter=on  N=100  InitialConditionSource=internal  InitialConditionForIntegrator=0  InitialConditionForFilter=0  DifferentiatorICPrevScaledInput=0  ExternalReset=none  TrackingMode=off  Kt=1  LimitOutput=on  UpperSaturationLimit=2  LowerSaturationLimit=-2  LinearizeAsGain=off  AntiWindupMode=none  Kb=1  POutMin=[]  POutMax=[]  IOutMin=[]  IOutMax=[]  DOutMin=[]  DOutMax=[]  NOutMin=[]  NOutMax=[]  SumOutMin=[]  SumOutMax=[]  SaturationOutMin=[]  SaturationOutMax=[]  PParamMin=[]  PParamMax=[]  IParamMin=[]  IParamMax=[]  DParamMin=[]  DParamMax=[]  NParamMin=[]  NParamMax=[]  KbParamMin=[]  KbParamMax=[]  KtParamMin=[]  KtParamMax=[]  KbOutMin=[]  KbOutMax=[]  KtOutMin=[]  KtOutMax=[]  IntegratorOutMin=[]  IntegratorOutMax=[]  FilterOutMin=[]  FilterOutMax=[]  SumI1OutMin=[]  SumI1OutMax=[]  SumI2OutMin=[]  SumI2OutMax=[]  SumI3OutMin=[]  SumI3OutMax=[]  SumDOutMin=[]  SumDOutMax=[]  DifferentiatorOutMin=[]  DifferentiatorOutMax=[]  IntegratorContinuousStateAttributes=''  IntegratorStateMustResolveToSignalObject=off  IntegratorRTWStateStorageClass=Auto  FilterContinuousStateAttributes=''  FilterStateMustResolveToSignalObject=off  FilterRTWStateStorageClass=Auto
  PI_Ireg1 : Scope
  Rtot_pu1 : Gain  Gain=Rtot_pu  SaturateOnIntegerOverflow=on  OutDataTypeStr=Inherit: Same as input  ParamDataTypeStr=Inherit: Same as input
  Rtot_pu5 : Gain  Gain=Rtot_pu  SaturateOnIntegerOverflow=on  OutDataTypeStr=Inherit: Same as input  ParamDataTypeStr=Inherit: Same as input
  Saturation : Saturate  UpperLimit=2  LowerLimit=-2
  Sum : Sum  Inputs=|-+
  VdVq_conv : Outport
  wires:
  Mux/1 -> PI_Ireg1/1, Add2/2
  PI/1 -> Add2/1  "PI"
  Sum/1 -> PI/1
  IdIq_ref/1 -> Sum/2, Demux1/1
  IdIq_mes/1 -> Sum/1
  Add2/1 -> Saturation/1
  Saturation/1 -> VdVq_conv/1
  VdVq_mes/1 -> Demux/1
  Demux/1 -> Add1/1
  Rtot_pu1/1 -> Add1/2
  Demux1/1 -> Rtot_pu1/1, Ltot_pu2/1
  Ltot_pu1/1 -> Add1/3
  Demux1/2 -> Ltot_pu1/1, Rtot_pu5/1
  Rtot_pu5/1 -> Add3/2
  Ltot_pu2/1 -> Add3/3
  Add1/1 -> Mux/1  "Feedforward"
  Demux/2 -> Add3/1
  Add3/1 -> Mux/2

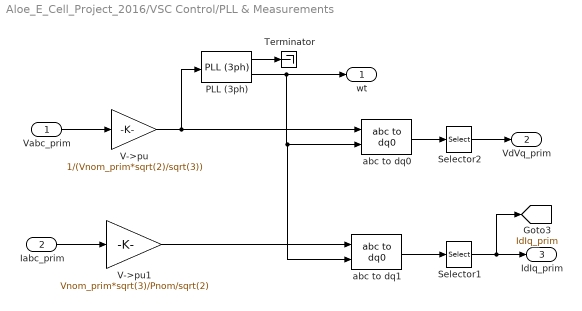
== system Aloe_E_Cell_Project_2016/VSC Control/PLL & Measurements ==
  Vabc_prim : Inport
  Iabc_prim : Inport  Port=2
  PLL (3ph) : powerlib_meascontrol/PLL/PLL (3ph)  Fmin=45  Par_Init="[-0.57  Fnom]"  ParK=[180, 3200, 1]  TcD=1e-4  MaxRateChangeFreq=12  FilterCutOffFreq=25  Ts=Ts  AGC=on
  Selector1 : Selector  InputPortWidth=3  IndexOptions=Index vector (dialog)  Indices=[1 2]  OutputSizes=1
  Selector2 : Selector  InputPortWidth=3  IndexOptions=Index vector (dialog)  Indices=[1 2]  OutputSizes=1
  Terminator : Terminator
  V->pu : Gain  Gain=1/(Vnom_prim*sqrt(2)/sqrt(3))  SaturateOnIntegerOverflow=on  OutDataTypeStr=Inherit: Same as input  ParamDataTypeStr=Inherit: Same as input
  V->pu1 : Gain  Gain=Vnom_prim*sqrt(3)/Pnom/sqrt(2)  SaturateOnIntegerOverflow=on  OutDataTypeStr=Inherit: Same as input  ParamDataTypeStr=Inherit: Same as input
  abc to dq0 : powerlib_meascontrol/Transformations/abc to dq0  Alignment=90 degrees behind phase A axis
  abc to dq1 : powerlib_meascontrol/Transformations/abc to dq0  Alignment=90 degrees behind phase A axis
  wt : Outport
  VdVq_prim : Outport  Port=2
  IdIq_prim : Outport  Port=3
  tag scope: IdIq_prim=global
  wires:
  V->pu1/1 -> abc to dq1/1
  V->pu/1 -> PLL (3ph)/1, abc to dq0/1
  abc to dq1/1 -> Selector1/1
  Vabc_prim/1 -> V->pu/1
  Iabc_prim/1 -> V->pu1/1
  abc to dq0/1 -> Selector2/1
  Selector2/1 -> VdVq_prim/1
  Selector1/1 -> [IdIq_prim], IdIq_prim/1
  PLL (3ph)/2 -> wt/1, abc to dq1/2, abc to dq0/2
  PLL (3ph)/1 -> Terminator/1

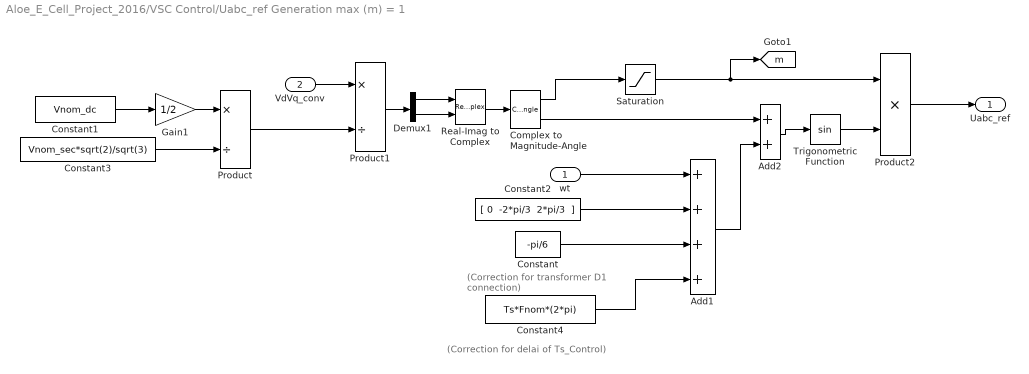
== system Aloe_E_Cell_Project_2016/VSC Control/Uabc_ref Generation max (m) = 1 ==
  note: (Correction for transformer
      |  D1 connection)
  note: (Correction for delai of Ts_Control)
  wt : Inport
  VdVq_conv : Inport  Port=2
  Add1 : Sum  Inputs=++++
  Add2 : Sum
  Complex to Magnitude-Angle : ComplexToMagnitudeAngle
  Constant : Constant  Value=-pi/6
  Constant1 : Constant  Value=Vnom_dc
  Constant2 : Constant  Value="[ 0  -2*pi/3  2*pi/3  ]"
  Constant3 : Constant  Value=Vnom_sec*sqrt(2)/sqrt(3)
  Constant4 : Constant  Value=Ts*Fnom*(2*pi)
  Demux1 : Demux  Outputs=2
  Gain1 : Gain  Gain=1/2
  Product : Product  Inputs=*/  RndMeth=Zero
  Product1 : Product  Inputs=*/  RndMeth=Zero
  Product2 : Product  Inputs=**  RndMeth=Zero
  Real-Imag to Complex : RealImagToComplex
  Saturation : Saturate  UpperLimit=1  LowerLimit=0
  Trigonometric Function : Trigonometry
  Uabc_ref : Outport
  tag scope: m=global
  wires:
  Complex to Magnitude-Angle/1 -> Saturation/1
  Constant1/1 -> Gain1/1
  VdVq_conv/1 -> Product1/1
  Product1/1 -> Demux1/1
  Gain1/1 -> Product/1
  Real-Imag to Complex/1 -> Complex to Magnitude-Angle/1
  Demux1/1 -> Real-Imag to Complex/1
  Demux1/2 -> Real-Imag to Complex/2
  Constant2/1 -> Add1/2
  Constant/1 -> Add1/3
  Constant3/1 -> Product/2
  Product/1 -> Product1/2
  Complex to Magnitude-Angle/2 -> Add2/1
  Add1/1 -> Add2/2
  Add2/1 -> Trigonometric Function/1
  Saturation/1 -> [m], Product2/1
  Trigonometric Function/1 -> Product2/2
  Product2/1 -> Uabc_ref/1
  wt/1 -> Add1/1
  Constant4/1 -> Add1/4

== system Aloe_E_Cell_Project_2016/VSC Control/VDC Regulator ==
  Vdc_mes : Inport  PortDimensions=1
  Vdc_ref : Inport  Port=2  PortDimensions=1
  PI : simulink/Continuous/PID Controller  Controller=PI  Form=Parallel  TimeDomain=Discrete-time  SampleTime=Ts  IntegratorMethod=Trapezoidal  FilterMethod=Forward Euler  ControllerParametersSource=internal  P=Kp_VDCreg  I=Ki_VDCreg  D=0  UseFilter=on  N=100  InitialConditionSource=internal  InitialConditionForIntegrator=0  InitialConditionForFilter=0  DifferentiatorICPrevScaledInput=0  ExternalReset=none  TrackingMode=off  Kt=1  LimitOutput=on  UpperSaturationLimit=1.5  LowerSaturationLimit=-1.5  LinearizeAsGain=off  AntiWindupMode=none  Kb=1  POutMin=[]  POutMax=[]  IOutMin=[]  IOutMax=[]  DOutMin=[]  DOutMax=[]  NOutMin=[]  NOutMax=[]  SumOutMin=[]  SumOutMax=[]  SaturationOutMin=[]  SaturationOutMax=[]  PParamMin=[]  PParamMax=[]  IParamMin=[]  IParamMax=[]  DParamMin=[]  DParamMax=[]  NParamMin=[]  NParamMax=[]  KbParamMin=[]  KbParamMax=[]  KtParamMin=[]  KtParamMax=[]  KbOutMin=[]  KbOutMax=[]  KtOutMin=[]  KtOutMax=[]  IntegratorOutMin=[]  IntegratorOutMax=[]  FilterOutMin=[]  FilterOutMax=[]  SumI1OutMin=[]  SumI1OutMax=[]  SumI2OutMin=[]  SumI2OutMax=[]  SumI3OutMin=[]  SumI3OutMax=[]  SumDOutMin=[]  SumDOutMax=[]  DifferentiatorOutMin=[]  DifferentiatorOutMax=[]  IntegratorContinuousStateAttributes=''  IntegratorStateMustResolveToSignalObject=off  IntegratorRTWStateStorageClass=Auto  FilterContinuousStateAttributes=''  FilterStateMustResolveToSignalObject=off  FilterRTWStateStorageClass=Auto
  Rtot_pu3 : Gain  Gain=1/Vnom_dc  SaturateOnIntegerOverflow=on  OutDataTypeStr=Inherit: Same as input  ParamDataTypeStr=Inherit: Same as input
  Sum : Sum  Inputs=|+-
  Id_ref : Outport  SampleTime=Ts  InitialOutput=0
  tag scope: Id_ref=global, Vdc_ref=global
  wires:
  Sum/1 -> Rtot_pu3/1
  Vdc_mes/1 -> Sum/1
  Vdc_ref/1 -> Sum/2, [Vdc_ref]
  Rtot_pu3/1 -> PI/1
  PI/1 -> [Id_ref], Id_ref/1
